simulink model "problem1"  (R2020b)
settings: Solver=VariableStepAuto  StartTime=0.0  StopTime=10.0  RelTol=1e-3
model workspace (MAT data in the model file):
  M1 = 100
  M2 = 4
  Var1 = 0
  b = 50
  k1 = 50
  k12 = 25
settings Model: Creator=admin  LastModifiedBy=admin

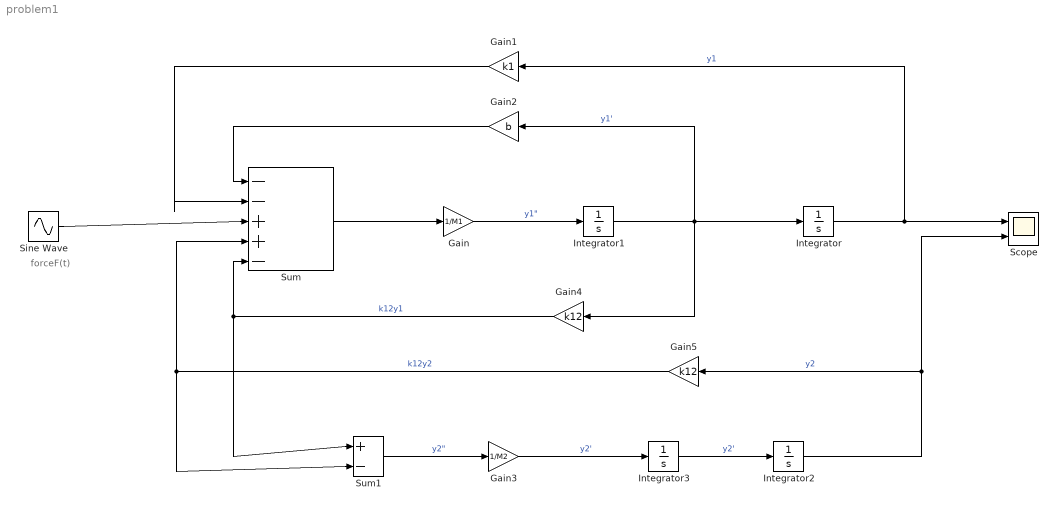
== system problem1 ==
  note: forceF(t)
  Gain : Gain  Gain=1/M1
  Gain1 : Gain  Gain=k1
  Gain2 : Gain  Gain=b
  Gain3 : Gain  Gain=1/M2
  Gain4 : Gain  Gain=k12
  Gain5 : Gain  Gain=k12
  Integrator{,1..3} (4 alike) : Integrator
  Scope : Scope  NumInputPorts=2
  Sine Wave : Sin  Amplitude=2  Frequency=10  SampleTime=0
  Sum : Sum  Inputs=|--++-
  Sum1 : Sum  Inputs=|+-
  wires:
  Gain1/1 -> Sum/2
  Gain2/1 -> Sum/1
  Sine Wave/1 -> Sum/3
  Gain/1 -> Integrator1/1  "y1\""
  Integrator1/1 -> Gain4/1, Gain2/1, Integrator/1  "y1'"
  Integrator3/1 -> Integrator2/1  "y2'"
  Gain3/1 -> Integrator3/1  "y2'"
  Sum1/1 -> Gain3/1  "y2\""
  Sum/1 -> Gain/1
  Gain5/1 -> Sum1/2, Sum/4  "k12y2"
  Gain4/1 -> Sum1/1, Sum/5  "k12y1"
  Integrator/1 -> Gain1/1, Scope/1  "y1"
  Integrator2/1 -> Gain5/1, Scope/2  "y2"
